simulink model "Sensors_and_actuators_ball_and_plate_2022b"  (R2022b)
settings: Solver=ode1  StartTime=0.0  StopTime=Inf  FixedStep=0.001  RelTol=1e-3
PostLoadFcn:
  | , if any(exist('dsrtsu_mdlpostloadfcn', 'file') ~= 0), dsrtsu_mdlpostloadfcn('Execute', bdroot); end,
InitFcn:
  | , if any(exist('rtifpga_mdlclblib', 'file') ~= 0), rtifpga_mdlclblib('Init', bdroot); end,
values from neighbouring files (symbols this model uses):
  a_y = ((0.1950)-(-0.1950))/(max_py-min_py)    [coordinate_transform.m]    (also in linearmap.m)
  b_x = -0.1950-(a_x*min_px)    [coordinate_transform.m]    (also in linearmap.m)
  b_y = -0.1950-(a_y*min_py)    [coordinate_transform.m]    (also in linearmap.m)
  center = cal1 + ((cal3-cal1)/2)    [coordinate_transform.m]    (also in linearmap.m)
libraries: rtiemclib x6, slpidlib x5, rtiethernetlib x3, rti1202lib_dac_class1 x3
(part 3 of 3)

== system Sensors_and_actuators_ball_and_plate_2022b/RTI Data/RTI Data Store/RTI Data Store ==
  RTI Data Store : Subsystem  mask(RTI_DATA_STORE){}
      mask help:
      | RTI Data Store Block. This block is used by RTI to store internal model dependent data. Deleting this block will result in data loss.
      |
      | NEVER DELETE, COPY, OR MODIFY THIS BLOCK!
      mask Help:
      | RTI Data Store Block. This block is used by RTI to store internal model dependent data. Deleting this block will result in data loss.
      | 
      | NEVER DELETE, COPY, OR MODIFY THIS BLOCK!
      mask Display: text(0.5, 0.5, ' ', 'HorizontalAlignment', 'center');

== system Sensors_and_actuators_ball_and_plate_2022b/RTI Data/RTI Data Store/RTI Data Store/RTI Data Store ==
  RTI Data Store : Subsystem  mask(RTI_DATA_STORE){}
      mask help:
      | RTI Data Store Block. This block is used by RTI to store internal model dependent data. Deleting this block will result in data loss.
      |
      | NEVER DELETE, COPY, OR MODIFY THIS BLOCK!
      mask Help:
      | RTI Data Store Block. This block is used by RTI to store internal model dependent data. Deleting this block will result in data loss.
      | 
      | NEVER DELETE, COPY, OR MODIFY THIS BLOCK!
      mask Display: text(0.5, 0.5, ' ', 'HorizontalAlignment', 'center');

== system Sensors_and_actuators_ball_and_plate_2022b/RTI Data/RTI Data Store/RTI Data Store/RTI Data Store/RTI Data Store ==

== matlab function Sensors_and_actuators_ball_and_plate_2022b/Inverse Kinematics/BoundsFunction1 ==
  data: ref input; outOfBounds output
function outOfBounds = fcn(ref)
    if ref > 0.06 || ref < 0
        outOfBounds = true;
    else
        outOfBounds = false;
    end
end

== matlab function Sensors_and_actuators_ball_and_plate_2022b/xy_controller/phi_saturation_check ==
  data: phi input; phi_saturation_reached output
function phi_saturation_reached = fcn(phi)
    if abs(phi) >= deg2rad(5)
        phi_saturation_reached = true;
    else
        phi_saturation_reached = false;
    end
end

== matlab function Sensors_and_actuators_ball_and_plate_2022b/Inverse Kinematics/Inverse Kinematics Calculation Function ==
  data: theta input; z1 output; phi input; z2 output; z3 output
function [z1, z2, z3] = fcn(theta, phi)
    d = 0.15; % [m]
    z1 = (-2*sqrt(3)/3) * d .* sin(theta);
    z2 = (sqrt(3)/3) * d .* sin(theta) - d .* cos(theta) .* sin(phi);
    z3 = (sqrt(3)/3) * d .* sin(theta) + d .* cos(theta) .* sin(phi);
end

== matlab function Sensors_and_actuators_ball_and_plate_2022b/Inverse Kinematics/BoundsFunction2 ==
  data: ref input; outOfBounds output
function outOfBounds = fcn(ref)
    if ref > 0.06 || ref < 0
        outOfBounds = true;
    else
        outOfBounds = false;
    end
end

== matlab function Sensors_and_actuators_ball_and_plate_2022b/Inverse Kinematics/BoundsFunction3 ==
  data: ref input; outOfBounds output
function outOfBounds = fcn(ref)
    if ref > 0.06 || ref < 0
        outOfBounds = true;
    else
        outOfBounds = false;
    end
end

== matlab function Sensors_and_actuators_ball_and_plate_2022b/Outputs to Amplifier1/MATLAB Function ==
  data: current input; saturation output
function saturation = fcn(current)
    if abs(current) >= 3
        saturation = true;
    else
        saturation = false;
    end
end

== matlab function Sensors_and_actuators_ball_and_plate_2022b/Outputs to Amplifier2/MATLAB Function ==
  data: current input; saturation output
function saturation = fcn(current)
    if abs(current) >= 3
        saturation = true;
    else
        saturation = false;
    end
end

== matlab function Sensors_and_actuators_ball_and_plate_2022b/Outputs to Amplifier3/MATLAB Function ==
  data: current input; saturation output
function saturation = fcn(current)
    if abs(current) >= 3
        saturation = true;
    else
        saturation = false;
    end
end

== matlab function Sensors_and_actuators_ball_and_plate_2022b/xy_controller/Integrator reset determination outer loop ==
  data: closed_loop_disabled input; integrator_reset input; Integrator_reset_mode_outerloop output
function Integrator_reset_mode_outerloop = fcn(closed_loop_disabled, integrator_reset)

    if integrator_reset == 1 || closed_loop_disabled == 0
        Integrator_reset_mode_outerloop = 1;
        return
    end
    
    Integrator_reset_mode_outerloop = 0;
end

== matlab function Sensors_and_actuators_ball_and_plate_2022b/Motor2/Integrator reset determination ==
  data: closed_loop_disabled input; integrator_reset input; Integrator_reset_mode_2 output
function Integrator_reset_mode_2 = fcn(closed_loop_disabled, integrator_reset)

    if integrator_reset == 1 || closed_loop_disabled == 0
        Integrator_reset_mode_2 = 1;
        return
    end
    
    Integrator_reset_mode_2 = 0;
end

== matlab function Sensors_and_actuators_ball_and_plate_2022b/Motor1/Integrator reset determination1 ==
  data: closed_loop_disabled input; integrator_reset input; Integrator_reset_mode_1 output
function Integrator_reset_mode_1 = fcn(closed_loop_disabled, integrator_reset)

    if integrator_reset == 1 || closed_loop_disabled == 0
        Integrator_reset_mode_1 = 1;
        return
    end
    
    Integrator_reset_mode_1 = 0;
end

== matlab function Sensors_and_actuators_ball_and_plate_2022b/Motor3/Integrator reset determination1 ==
  data: closed_loop_disabled input; integrator_reset input; Integrator_reset_mode_3 output
function Integrator_reset_mode_3 = fcn(closed_loop_disabled, integrator_reset)

    if integrator_reset == 1 || closed_loop_disabled == 0
        Integrator_reset_mode_3 = 1;
        return
    end
    
    Integrator_reset_mode_3 = 0;
end

== matlab function Sensors_and_actuators_ball_and_plate_2022b/xy_controller/theta_saturation_check ==
  data: theta input; theta_saturation_reached output
function theta_saturation_reached = fcn(theta)
    if abs(theta) >= deg2rad(5)
        theta_saturation_reached = true;
    else
        theta_saturation_reached = false;
    end
end
